simulink subsystem "Task_Controls_ThorneFleissner"  (R2020b)
settings: Solver=VariableStepAuto  StartTime=0.0  StopTime=10.0  RelTol=1e-3
libraries: simulink_extras x3
settings Model: Creator=rthom  LastModifiedBy=rthom

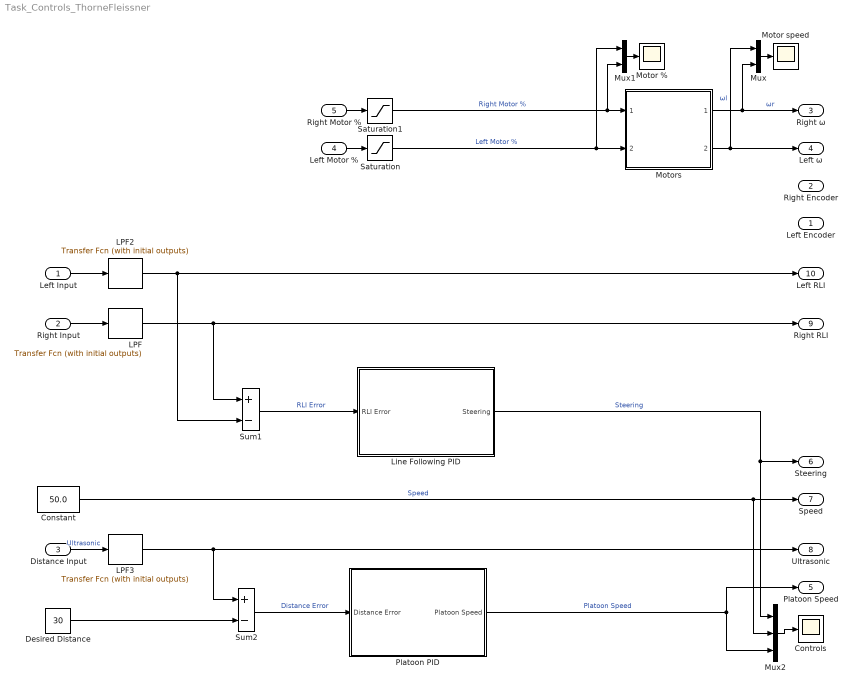
== system Task_Controls_ThorneFleissner ==
  Left Input : Inport
  Right Input : Inport  Port=2
  Distance Input : Inport  Port=3
  Left Motor % : Inport  Port=4
  Right Motor % : Inport  Port=5
  Constant : Constant  Value=50.0
  Controls : Scope
  Desired Distance : Constant  Value=30
  LPF : simulink_extras/Additional Linear/Transfer Fcn (with initial outputs)  N=[1]  D="[0.02  1]"  Y0=0  U0=0
  LPF2 : simulink_extras/Additional Linear/Transfer Fcn (with initial outputs)  N=[1]  D="[0.02  1]"  Y0=0  U0=0
  LPF3 : simulink_extras/Additional Linear/Transfer Fcn (with initial outputs)  N=[1]  D="[0.02  1]"  Y0=0  U0=0
  Line Following PID : Subsystem
  Motor % : Scope
  Motor speed : Scope
  Motors : Subsystem  ReferencedSubsystem=Motors_ThorneFleissner
  Mux : Mux  Inputs=2
  Mux1 : Mux  Inputs=2
  Mux2 : Mux  Inputs=3
  Platoon PID : Subsystem
  Saturation : Saturate  UpperLimit=100  LowerLimit=-100
  Saturation1 : Saturate  UpperLimit=100  LowerLimit=-100
  Sum1 : Sum  Inputs=+-
  Sum2 : Sum  Inputs=+-
  Left Encoder : Outport
  Right Encoder : Outport  Port=2
  Right ω : Outport  Port=3
  Left ω : Outport  Port=4
  Platoon Speed : Outport  Port=5
  Steering : Outport  Port=6
  Speed : Outport  Port=7
  Ultrasonic : Outport  Port=8
  Right RLI : Outport  Port=9
  Left RLI : Outport  Port=10
  wires:
  LPF2/1 -> Left RLI/1, Sum1/2
  Motors/1 -> Right ω/1, Mux/2  "ωr"
  Motors/2 -> Left ω/1, Mux/1  "ωl"
  Mux/1 -> Motor speed/1
  Mux1/1 -> Motor %/1
  Saturation1/1 -> Mux1/2, Motors/1  "Right Motor %"
  Saturation/1 -> Mux1/1, Motors/2  "Left Motor %"
  Constant/1 -> Speed/1, Mux2/2  "Speed"
  Left Motor %/1 -> Saturation/1
  Right Motor %/1 -> Saturation1/1
  Mux2/1 -> Controls/1
  Right Input/1 -> LPF/1
  LPF/1 -> Right RLI/1, Sum1/1
  Left Input/1 -> LPF2/1
  Distance Input/1 -> LPF3/1  "Ultrasonic"
  Desired Distance/1 -> Sum2/2
  LPF3/1 -> Ultrasonic/1, Sum2/1
  Platoon PID/1(Platoon Speed) -> Platoon Speed/1, Mux2/3  "Platoon Speed"
  Sum2/1 -> Platoon PID/1(Distance Error)  "Distance Error"
  Line Following PID/1(Steering) -> Steering/1, Mux2/1  "Steering"
  Sum1/1 -> Line Following PID/1(RLI Error)  "RLI Error"

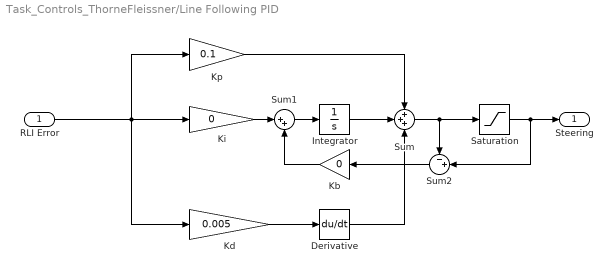
== system Task_Controls_ThorneFleissner/Line Following PID ==
  RLI Error : Inport
  Derivative : Derivative
  Integrator : Integrator
  Kb : Gain  Gain=0
  Kd : Gain  Gain=0.005
  Ki : Gain  Gain=0
  Kp : Gain  Gain=0.1
  Saturation : Saturate  UpperLimit=15  LowerLimit=-15
  Sum : Sum  Inputs=+++
  Sum1 : Sum  Inputs=|++
  Sum2 : Sum  Inputs=-+|
  Steering : Outport
  wires:
  Sum2/1 -> Kb/1
  Kb/1 -> Sum1/2
  Sum1/1 -> Integrator/1
  Ki/1 -> Sum1/1
  Saturation/1 -> Steering/1, Sum2/2
  Derivative/1 -> Sum/3
  RLI Error/1 -> Kp/1, Ki/1, Kd/1
  Integrator/1 -> Sum/2
  Kp/1 -> Sum/1
  Kd/1 -> Derivative/1
  Sum/1 -> Saturation/1, Sum2/1

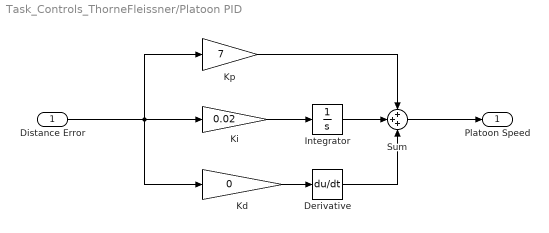
== system Task_Controls_ThorneFleissner/Platoon PID ==
  Distance Error : Inport
  Derivative : Derivative
  Integrator : Integrator
  Kd : Gain  Gain=0
  Ki : Gain  Gain=0.02
  Kp : Gain  Gain=7
  Sum : Sum  Inputs=+++
  Platoon Speed : Outport
  wires:
  Derivative/1 -> Sum/3
  Distance Error/1 -> Kp/1, Ki/1, Kd/1
  Integrator/1 -> Sum/2
  Ki/1 -> Integrator/1
  Kp/1 -> Sum/1
  Kd/1 -> Derivative/1
  Sum/1 -> Platoon Speed/1
